simulink model "MPCmodual2O"  (R2015b)
settings: Solver=ode4  StartTime=0.0  StopTime=200  FixedStep=Ts  RelTol=1e-3
values from neighbouring files (symbols this model uses):
  Ts = 0.01    [MOSA_mpc_sim.m]    (also in MPC1DOF_disturbance_unkonwn.m = 0.0125; MPC1DOF_disurbance_known.m = 0.0125; MPC5DOFLinear.m = 0.0125; MPCLinear2O.m = 0.0125)
undefined symbols (not defined in the file or in its folder): Am, Bm, Cm, Dm, sigbuilder_block
libraries: mpclib x1
settings Model: Creator=yuy13010  LastModifiedBy=yuy13010

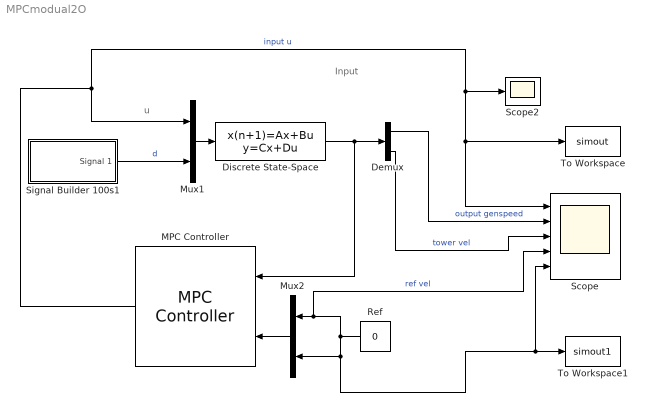
== system MPCmodual2O ==
  note: u
  note: Input
  Demux : Demux  Outputs=2
  Discrete State-Space : DiscreteStateSpace  A=Am  B=Bm  C=Cm  D=Dm  SampleTime=Ts
  MPC Controller : mpclib/MPC Controller  SCDEnableBlockLinearizationSpecification=on  mpcobj=mpcobj  x0=[]  is_multiple=0  enable_value=0  return_u0=off  ref_from_ws=off  ref_signal_name=[]  ref_preview=off  md_from_ws=off  md_signal_name=[]  md_preview=off  from_project=off  project_file=MPCtask.mat  md_inport=off  mv_inport=off  cost_outport=off  return_sequence=off  return_qpstatus=off  return_state=off  state_inport=off  lims_inport=off  ywt_inport=off  is_designfromscratch=0  uwt_inport=off  duwt_inport=off  rhoeps_inport=off  uref_inport=off  n_ts=0.0125  n_mv=1  n_md=0  n_ud=0  n_mo=2  n_uo=0  BlockDataType=double  SampleTimeInherited=off  switch_inport=off
  Mux1 : Mux  Inputs=2
  Mux2 : Mux  Inputs=2
  Ref : Constant  Value=0
  Scope : Scope  NumInputPorts=5
  Scope2 : Scope
  Signal Builder 100s1 : Subsystem  Tag=STV Subsys  LoadFcn=sigbuilder_block('load');  StartFcn=sigbuilder_block('start');  StopFcn=sigbuilder_block('stop');  ClipboardFcn=sigbuilder_block('clipboard');  mask(Sigbuilder block){}
      mask help: Simulink:masks:SigbuilderBlock_MD
      mask init:
      | if ~strcmp(get_param(bdroot(gcbh),'SimulationStatus'),'stopped') tuvar = sigbuilder_block('maskInit'); end
      settings: CopyFcn=sigbuilder_block('copy');  DeleteFcn=sigbuilder_block('delete');  ModelCloseFcn=sigbuilder_block('modelClose');  PreSaveFcn=sigbuilder_block('preSave');  PauseFcn=sigbuilder_block('pause');  ContinueFcn=sigbuilder_block('continue');  NameChangeFcn=sigbuilder_block('namechange');  OpenFcn=sigbuilder_block('open',[5.4 15 757.2 461.4 ]);  CloseFcn=sigbuilder_block('close');
      mask Display: plot(0, 0, 100, 100,[2, 2, 32, 32, 2], [68, 8, 8, 68, 68],[32, 2], [38, 38], [32, 19, 2],[53, 60, 44], [32, 17, 17, 2],[16, 16, 31, 31]);txt = getActiveGroup(gcbh);text(2, 100, txt,'verticalAlignment', 'top');
  To Workspace : ToWorkspace  VariableName=simout  SaveFormat=Timeseries  SampleTime=-1
  To Workspace1 : ToWorkspace  VariableName=simout1  SaveFormat=Timeseries  SampleTime=-1
  wires:
  Ref/1 -> Mux2/2, Scope/5, To Workspace1/1, Scope/4, Mux2/1  "ref vel"
  Mux1/1 -> Discrete State-Space/1
  Signal Builder 100s1/1(Signal 1) -> Mux1/2  "d"
  Mux2/1 -> MPC Controller/2
  Discrete State-Space/1 -> MPC Controller/1, Demux/1
  Demux/1 -> Scope/2  "output genspeed"
  MPC Controller/1 -> Mux1/1, Scope/1, To Workspace/1, Scope2/1  "input u"
  Demux/2 -> Scope/3  "tower vel"

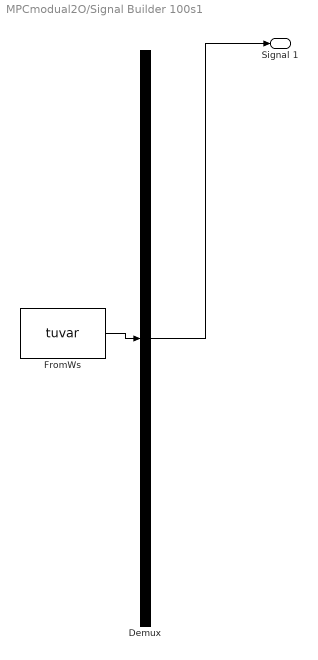
== system MPCmodual2O/Signal Builder 100s1 ==
  Demux : Demux  Tag=STV Demux  Outputs=1
  FromWs : FromWorkspace  Tag=STV FromWs  VariableName=tuvar  SampleTime=0
      SigBuilderData=|
      | common.afterFinalStr = 'Extrapolate'
      | common.sampleTime = 0
      | dataSet.timeRange = [0 100]
      | dataSet.name = 'Group 1'
      | sbobj.Groups.Name = 'Group 1'
      | sbobj.Groups.Signals.Name = 'Signal 1'
      | sbobj.Groups.Signals.XData = [0 19.95 19.95 40 40 60 60 79.8 79.8 100]
      | sbobj.Groups.Signals.YData = [1.9 1.9 3.95 3.95 8 8 12 12 16 16]
      | sbobj.Groups.TimeRange = [0 100]
  Signal 1 : Outport  Tag=STV Outport
  wires:
  FromWs/1 -> Demux/1
  Demux/1 -> Signal 1/1
